simulink model "QueueSortingPoliciesModel_org"  (Simulink 10.0)
settings: Solver=VariableStepAuto  StartTime=0.0  StopTime=10.0  RelTol=1e-3
libraries: simulink x1
settings Model: Creator=The MathWorks, Inc.  LastModifiedBy=bhisma
settings DataIOCC: SaveFormat=Dataset  ReturnWorkspaceOutputs=on
settings OptimizationCC: LifeSpan=auto
settings DebuggingCC: UnderspecifiedInitializationDetection=Simplified  MergeDetectMultiDrivingBlocksExec=error  SFUnexpectedBacktrackingDiag=error  SFNoUnconditionalDefaultTransitionDiag=error  SFExecutionAtInitializationDiag=warning  ArithmeticOperatorsInVariantConditions=error
settings HardwareCC: ProdBitPerPointer=64  ProdBitPerSizeT=64  ProdBitPerPtrDiffT=64  ProdLargestAtomicFloat=Float  ProdIntDivRoundTo=Zero  ProdEndianess=LittleEndian  ProdWordSize=64  ProdHWDeviceType=Intel->x86-64 (Windows64)
settings ModelReferenceCC: PropagateSignalLabelsOutOfModel=on
settings SFSimCC: SimUseLocalCustomCode=on  CustomCodeUndefinedFunction=FilterOut
settings RTWCC: RTWUseLocalCustomCode=on
settings CodeAppCC: StateflowObjectComments=off
settings GRTTargetCC: TargetLangStandard=C99 (ISO)  CombineOutputUpdateFcns=on  GRTInterface=off
settings ConfigComp: CovMetricSettings=dwe  CovHtmlReporting=off  CovSaveCumulativeToWorkspaceVar=off  CovSaveSingleToWorkspaceVar=off

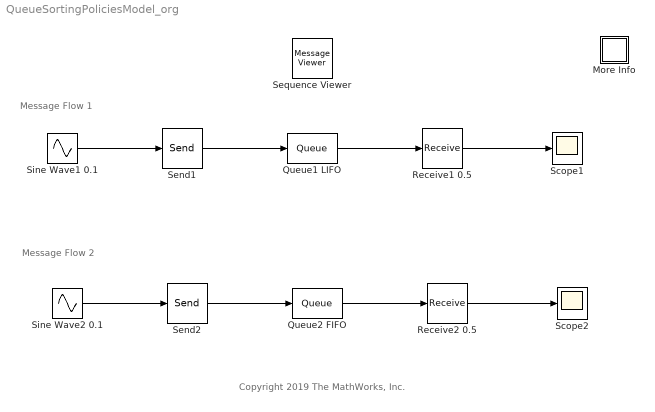
== system QueueSortingPoliciesModel_org ==
  note: Message Flow 2
  note: Message Flow 1
  note: Copyright 2019 The MathWorks, Inc.
  More Info : Subsystem
      settings: OpenFcn=showExample('simulink/UseAQueueBlockToManageMessagesExample')
      mask Display: disp('?')
  Queue1 LIFO : Queue  InputPortMessageModes=m  OutputPortMessageModes=m  OverwriteOldest=on  Capacity=100  QueueType=LIFO
  Queue2 FIFO : Queue  InputPortMessageModes=m  OutputPortMessageModes=m  OverwriteOldest=on  Capacity=100
  Receive1 0.5 : Receive  InputPortMessageModes=m  UseInternalQueue=off  QueueOverwriting=on  QueueLength=1  QueueType=LIFO  SampleTime=0.5
  Receive2 0.5 : Receive  InputPortMessageModes=m  UseInternalQueue=off  QueueOverwriting=on  QueueLength=1  QueueType=LIFO  SampleTime=0.5
  Scope1 : Scope
  Scope2 : Scope
  Send1 : Send  OutputPortMessageModes=m
  Send2 : Send  OutputPortMessageModes=m
  Sequence Viewer : MessageViewer  History=1000  SavedRootId=#
  Sine Wave1 0.1 : Sin  SampleTime=0.1
  Sine Wave2 0.1 : Sin  SampleTime=0.1
  wires:
  Receive2 0.5/1 -> Scope2/1
  Send2/1 -> Queue2 FIFO/1
  Queue2 FIFO/1 -> Receive2 0.5/1
  Receive1 0.5/1 -> Scope1/1
  Send1/1 -> Queue1 LIFO/1
  Queue1 LIFO/1 -> Receive1 0.5/1
  Sine Wave1 0.1/1 -> Send1/1
  Sine Wave2 0.1/1 -> Send2/1

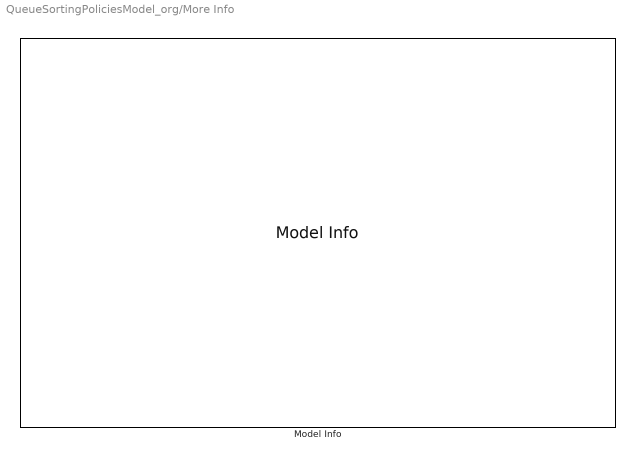
== system QueueSortingPoliciesModel_org/More Info ==
  Model Info : simulink/Model-Wide Utilities/Model Info  Frame=on  DisplayStringWithTags=|  HorizontalTextAlignment=Left  LeftAlignmentValue=0.02
      | Model Description:
      | -------------------
      | This example shows how to use the Message Delay block to model a variable
      | speed conveyor belt between two airport terminals. The passengers step on
      | the conveyor belt following a Poisson distribution. Since passengers are
      | discrete entities, they are naturally modeled by Simulink(R) messages,
      | which are created by the Entity Generator block. When a passenger, i.e.,
      | a Simulink(R) message, is sent to the Message Delay block, the block
      | will hold it until it arrives at the other end of the conveyor belt. The
      | length of the delay time is automatically calculated by Simulink(R) based
      | on the ETA (estimated time of arrival), which is calculated by the
      | Stateflow(R) Chart. The operation of the conveyor belt depends on the
      | load and its transfer characteristics.
